simulink library "csc_lc_limit_check_lib"  (R2014b)
settings: Solver=ode45  StartTime=0.0  StopTime=10.0  RelTol=1e-3
undefined symbols (not defined in the file or in its folder): csc_sc_dt, lc_ap_default_states
libraries: util_info_lib x1, csc_apc_actionpoint_collection_lib x1, csc_wpc_watchpoint_collection_lib x1, csu_elc_execute_lc_commands_lib x1
settings Model: Creator=mstewart  LastModifiedBy=mstewart

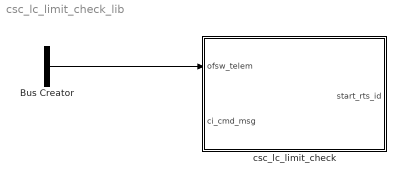
== system csc_lc_limit_check_lib ==
  Bus Creator : BusCreator  Inputs=2  OutDataTypeStr=Bus: sch_bus_msg  NonVirtualBus=on
  csc_lc_limit_check : Subsystem  TreatAsAtomicUnit=on  SystemSampleTime=csc_sc_dt
  wires:
  Bus Creator/1 -> csc_lc_limit_check/1(ofsw_telem)
  ? -> Bus Creator/1  "met_mseconds"
  ? -> Bus Creator/2  "met_seconds"

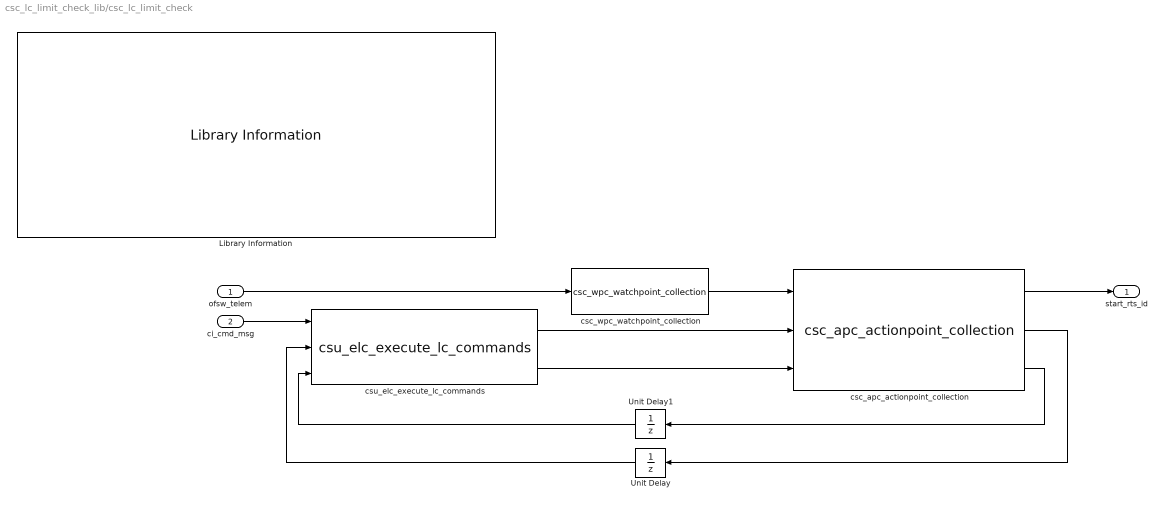
== system csc_lc_limit_check_lib/csc_lc_limit_check ==
  ofsw_telem : Inport
  ci_cmd_msg : Inport  Port=2  OutDataTypeStr=Bus: ci_cmd_msg
  Library Information : util_info_lib/Library Information  owner='escrane'
  Unit Delay : UnitDelay  InitialCondition=lc_ap_default_states  SampleTime=-1
  Unit Delay1 : UnitDelay  SampleTime=-1
  csc_apc_actionpoint_collection : csc_apc_actionpoint_collection_lib/csc_apc_actionpoint_collection  SystemSampleTime=-1
  csc_wpc_watchpoint_collection : csc_wpc_watchpoint_collection_lib/csc_wpc_watchpoint_collection  SystemSampleTime=-1
  csu_elc_execute_lc_commands : csu_elc_execute_lc_commands_lib/csu_elc_execute_lc_commands
  start_rts_id : Outport
  wires:
  Unit Delay1/1 -> csu_elc_execute_lc_commands/3
  Unit Delay/1 -> csu_elc_execute_lc_commands/2
  ci_cmd_msg/1 -> csu_elc_execute_lc_commands/1
  ofsw_telem/1 -> csc_wpc_watchpoint_collection/1
  csc_wpc_watchpoint_collection/1 -> csc_apc_actionpoint_collection/1
  csu_elc_execute_lc_commands/1 -> csc_apc_actionpoint_collection/2
  csu_elc_execute_lc_commands/2 -> csc_apc_actionpoint_collection/3
  csc_apc_actionpoint_collection/3 -> Unit Delay1/1
  csc_apc_actionpoint_collection/2 -> Unit Delay/1
  csc_apc_actionpoint_collection/1 -> start_rts_id/1
